simulink model "SIMULINK_U_a_C"  (R2023b)
settings: Solver=FixedStepAuto  StartTime=0.0  StopTime=sim_end_time  FixedStep=fixed_step_size  RelTol=1e-3
undefined symbols (not defined in the file): a, act_end, b, battery_threshold, bb, draw_gif, droneyeeUAV2_NUM, droneyeeUAV3_NUM, droneyeeUAV4_NUM, droneyeeUAV5_NUM, fixed_step_size, k, KD_x, KD_y, kd_z, KDD_x, KDD_y, KI_x, KI_y, ki_z, KII_x, KII_y, KP_x, KP_y, kp_z, KPP_x, KPP_y, lmt, omega, R, sim_end_time, uav10num, uav1num, uav2num, uav3num, uav4num, uav5num, uav6num, uav7num, uav8num, uav9num, UAV_NUM, Vel_Switch_1, Vel_Switch_10, Vel_Switch_11, Vel_Switch_12, Vel_Switch_13, Vel_Switch_14, Vel_Switch_15, Vel_Switch_16, Vel_Switch_17, Vel_Switch_18, Vel_Switch_19, Vel_Switch_2, Vel_Switch_20, Vel_Switch_3, Vel_Switch_4, Vel_Switch_5, Vel_Switch_6, Vel_Switch_7 ... (+11)
libraries: simulink x120, aerolibanimutils x1
(part 5 of 10)

== system SIMULINK_U_a_C/CMD_car1/CMD6 ==
  "clock " : Inport
  droneyeeUAV_states : Inport  Port=2
  droneyeeUAV_bat : Inport  Port=3
  Bus Selector : BusSelector  OutputSignals=x,y,z
  Constant : Constant  Value=sim_end_time
  Constant1 : Constant  Value=battery_threshold
  Constant2 : Constant  Value=z_d_for_land
  Constant3 : Constant  Value=0
  Constant4 : Constant  Value=UAV_NUM
  MATLAB Function1 : MATLAB Function  TreatAsAtomicUnit=on
  Manual Switch2 : ManualSwitch
  Sine Wave2 : Sin  Amplitude=0.3  Frequency=1.0
  Slider Gain3 : simulink/Math Operations/Slider Gain  gain=1  low=0  high=2
  Subsystem : Subsystem
  x_d : Outport  VectorParamsAs1DForOutWhenUnconnected=off
  y_d : Outport  Port=2  VectorParamsAs1DForOutWhenUnconnected=off
  z_d : Outport  Port=3  VectorParamsAs1DForOutWhenUnconnected=off
  yaw_d : Outport  Port=4  VectorParamsAs1DForOutWhenUnconnected=off
  wires:
  Manual Switch2/1 -> Slider Gain3/1
  Slider Gain3/1 -> yaw_d/1
  Sine Wave2/1 -> Manual Switch2/2
  Constant3/1 -> Manual Switch2/1
  MATLAB Function1/2(y_d_) -> y_d/1
  Constant2/1 -> MATLAB Function1/11(z_d_for_land)
  Subsystem/3(zd) -> MATLAB Function1/3(z_d)
  Constant1/1 -> MATLAB Function1/10(battery_threshold)
  MATLAB Function1/3(z_d_) -> z_d/1
  droneyeeUAV_states/1 -> Subsystem/2(uavstates), Bus Selector/1
  MATLAB Function1/1(x_d_) -> x_d/1
  Constant4/1 -> MATLAB Function1/12(UAV_NUM)
  Constant/1 -> MATLAB Function1/9(sim_time_end)
  Subsystem/1("xd ") -> MATLAB Function1/1(x_d)
  Subsystem/2(yd) -> MATLAB Function1/2(y_d)
  "clock "/1 -> Subsystem/1(clock), MATLAB Function1/4(timestamp)
  droneyeeUAV_bat/1 -> MATLAB Function1/8(battery_status)
  Bus Selector/1 -> MATLAB Function1/5(x)  "<x>"
  Bus Selector/2 -> MATLAB Function1/6(y)  "<y>"
  Bus Selector/3 -> MATLAB Function1/7(z)  "<z>"

== system SIMULINK_U_a_C/CMD_car1/CMD7 ==
  "clock " : Inport
  droneyeeUAV_states : Inport  Port=2
  droneyeeUAV_bat : Inport  Port=3
  Bus Selector : BusSelector  OutputSignals=x,y,z
  Constant : Constant  Value=sim_end_time
  Constant1 : Constant  Value=battery_threshold
  Constant2 : Constant  Value=z_d_for_land
  Constant3 : Constant  Value=0
  Constant4 : Constant  Value=UAV_NUM
  MATLAB Function1 : MATLAB Function  TreatAsAtomicUnit=on
  Manual Switch2 : ManualSwitch
  Sine Wave2 : Sin  Amplitude=0.3  Frequency=1.0
  Slider Gain3 : simulink/Math Operations/Slider Gain  gain=1  low=0  high=2
  Subsystem : Subsystem
  Terminator : Terminator
  x_d : Outport  VectorParamsAs1DForOutWhenUnconnected=off
  y_d : Outport  Port=2  VectorParamsAs1DForOutWhenUnconnected=off
  z_d : Outport  Port=3  VectorParamsAs1DForOutWhenUnconnected=off
  yaw_d : Outport  Port=4  VectorParamsAs1DForOutWhenUnconnected=off
  wires:
  Manual Switch2/1 -> Slider Gain3/1
  Slider Gain3/1 -> yaw_d/1
  Sine Wave2/1 -> Manual Switch2/2
  Constant3/1 -> Manual Switch2/1
  Bus Selector/1 -> MATLAB Function1/5(x)  "<x>"
  MATLAB Function1/2(y_d_) -> y_d/1
  Constant2/1 -> MATLAB Function1/11(z_d_for_land)
  Subsystem/3(zd) -> MATLAB Function1/3(z_d)
  Bus Selector/2 -> MATLAB Function1/6(y)  "<y>"
  Constant1/1 -> MATLAB Function1/10(battery_threshold)
  MATLAB Function1/3(z_d_) -> z_d/1
  MATLAB Function1/1(x_d_) -> x_d/1
  Constant4/1 -> MATLAB Function1/12(UAV_NUM)
  Bus Selector/3 -> MATLAB Function1/7(z)  "<z>"
  Constant/1 -> MATLAB Function1/9(sim_time_end)
  Subsystem/1("xd ") -> MATLAB Function1/1(x_d)
  Subsystem/2(yd) -> MATLAB Function1/2(y_d)
  "clock "/1 -> Subsystem/1(clock), MATLAB Function1/4(timestamp)
  droneyeeUAV_bat/1 -> MATLAB Function1/8(battery_status)
  droneyeeUAV_states/1 -> Subsystem/2(uavstates), Bus Selector/1

== system SIMULINK_U_a_C/CMD_car1/CMD8 ==
  "clock " : Inport
  droneyeeUAV_states : Inport  Port=2
  droneyeeUAV_bat : Inport  Port=3
  Bus Selector : BusSelector  OutputSignals=x,y,z
  Constant : Constant  Value=sim_end_time
  Constant1 : Constant  Value=battery_threshold
  Constant2 : Constant  Value=z_d_for_land
  Constant3 : Constant  Value=0
  Constant4 : Constant  Value=UAV_NUM
  MATLAB Function1 : MATLAB Function  TreatAsAtomicUnit=on
  Manual Switch2 : ManualSwitch
  Sine Wave2 : Sin  Amplitude=0.3  Frequency=1.0
  Slider Gain3 : simulink/Math Operations/Slider Gain  gain=1  low=0  high=2
  Subsystem : Subsystem
  x_d : Outport  VectorParamsAs1DForOutWhenUnconnected=off
  y_d : Outport  Port=2  VectorParamsAs1DForOutWhenUnconnected=off
  z_d : Outport  Port=3  VectorParamsAs1DForOutWhenUnconnected=off
  yaw_d : Outport  Port=4  VectorParamsAs1DForOutWhenUnconnected=off
  wires:
  Manual Switch2/1 -> Slider Gain3/1
  Slider Gain3/1 -> yaw_d/1
  Sine Wave2/1 -> Manual Switch2/2
  Constant3/1 -> Manual Switch2/1
  MATLAB Function1/2(y_d_) -> y_d/1
  Constant2/1 -> MATLAB Function1/11(z_d_for_land)
  Subsystem/3(zd) -> MATLAB Function1/3(z_d)
  Constant1/1 -> MATLAB Function1/10(battery_threshold)
  MATLAB Function1/3(z_d_) -> z_d/1
  droneyeeUAV_states/1 -> Subsystem/2(uavstates), Bus Selector/1
  MATLAB Function1/1(x_d_) -> x_d/1
  Constant4/1 -> MATLAB Function1/12(UAV_NUM)
  Constant/1 -> MATLAB Function1/9(sim_time_end)
  Subsystem/1("xd ") -> MATLAB Function1/1(x_d)
  Subsystem/2(yd) -> MATLAB Function1/2(y_d)
  "clock "/1 -> Subsystem/1(clock), MATLAB Function1/4(timestamp)
  droneyeeUAV_bat/1 -> MATLAB Function1/8(battery_status)
  Bus Selector/1 -> MATLAB Function1/5(x)  "<x>"
  Bus Selector/2 -> MATLAB Function1/6(y)  "<y>"
  Bus Selector/3 -> MATLAB Function1/7(z)  "<z>"

== system SIMULINK_U_a_C/CMD_car1/CMD9 ==
  "clock " : Inport
  droneyeeUAV_states : Inport  Port=2
  droneyeeUAV_bat : Inport  Port=3
  Bus Selector : BusSelector  OutputSignals=x,y,z
  Constant : Constant  Value=sim_end_time
  Constant1 : Constant  Value=battery_threshold
  Constant2 : Constant  Value=z_d_for_land
  Constant3 : Constant  Value=0
  Constant4 : Constant  Value=UAV_NUM
  MATLAB Function1 : MATLAB Function  TreatAsAtomicUnit=on
  Manual Switch2 : ManualSwitch
  Sine Wave2 : Sin  Amplitude=0.3  Frequency=1.0
  Slider Gain3 : simulink/Math Operations/Slider Gain  gain=1  low=0  high=2
  Subsystem : Subsystem
  Terminator : Terminator
  x_d : Outport  VectorParamsAs1DForOutWhenUnconnected=off
  y_d : Outport  Port=2  VectorParamsAs1DForOutWhenUnconnected=off
  z_d : Outport  Port=3  VectorParamsAs1DForOutWhenUnconnected=off
  yaw_d : Outport  Port=4  VectorParamsAs1DForOutWhenUnconnected=off
  wires:
  Manual Switch2/1 -> Slider Gain3/1
  Slider Gain3/1 -> yaw_d/1
  Sine Wave2/1 -> Manual Switch2/2
  Constant3/1 -> Manual Switch2/1
  Bus Selector/1 -> MATLAB Function1/5(x)  "<x>"
  MATLAB Function1/2(y_d_) -> y_d/1
  Constant2/1 -> MATLAB Function1/11(z_d_for_land)
  Subsystem/3(zd) -> MATLAB Function1/3(z_d)
  Bus Selector/2 -> MATLAB Function1/6(y)  "<y>"
  Constant1/1 -> MATLAB Function1/10(battery_threshold)
  MATLAB Function1/3(z_d_) -> z_d/1
  MATLAB Function1/1(x_d_) -> x_d/1
  Constant4/1 -> MATLAB Function1/12(UAV_NUM)
  Bus Selector/3 -> MATLAB Function1/7(z)  "<z>"
  Constant/1 -> MATLAB Function1/9(sim_time_end)
  Subsystem/1("xd ") -> MATLAB Function1/1(x_d)
  Subsystem/2(yd) -> MATLAB Function1/2(y_d)
  "clock "/1 -> Subsystem/1(clock), MATLAB Function1/4(timestamp)
  droneyeeUAV_bat/1 -> MATLAB Function1/8(battery_status)
  droneyeeUAV_states/1 -> Subsystem/2(uavstates), Bus Selector/1

== system SIMULINK_U_a_C/control system_UAV/Baseline Controller1 ==
  X_e : Inport
  Y_e : Inport  Port=2
  " Z_e " : Inport  Port=3
  Yaw_e : Inport  Port=4
  " V_x" : Inport  Port=5
  V_y : Inport  Port=6
  "V_z " : Inport  Port=7
  x_d : Inport  Port=8
  y_d : Inport  Port=9
  Z_d : Inport  Port=10
  Yaw_d : Inport  Port=11
  Constant : Constant  Commented=on  Value=omega*R*2
  Demux : Demux  Outputs=2
  Heading controller : Subsystem
  "Height controller " : Subsystem
  MATLAB Function : MATLAB Function  Commented=on  TreatAsAtomicUnit=on
  Position controller : Subsystem
  Saturation1 : Saturate  UpperLimit=lmt  LowerLimit=-lmt
  Saturation2 : Saturate  UpperLimit=lmt  LowerLimit=-lmt
  ux : Outport  VectorParamsAs1DForOutWhenUnconnected=off
  uy : Outport  Port=2  VectorParamsAs1DForOutWhenUnconnected=off
  Z_velocity_d. [-1,1] : Outport  Port=3  VectorParamsAs1DForOutWhenUnconnected=off
  yaw_rate_d [-1,1] : Outport  Port=4  VectorParamsAs1DForOutWhenUnconnected=off
  wires:
  " Z_e "/1 -> "Height controller "/2(Z_e (m))
  X_e/1 -> Position controller/1(X_e (m))
  Y_e/1 -> Position controller/2(Y_e (m))
  Yaw_d/1 -> Heading controller/2(yaw_d. (rad))
  Demux/1 -> ux/1
  Demux/2 -> uy/1
  Constant/1 -> MATLAB Function/2(a)
  Z_d/1 -> "Height controller "/1(Z_d. (m))
  x_d/1 -> Position controller/3(X_d (m))
  y_d/1 -> Position controller/4(Y_d (m))
  Yaw_e/1 -> Heading controller/1(yaw_e (rad))  "yaw"
  "V_z "/1 -> "Height controller "/3(V_z)
  Heading controller/1(yaw_rate_d. (rad/s)) -> yaw_rate_d [-1,1]/1
  "Height controller "/1(Z_velocity_d (m/s)) -> Saturation2/1
  Saturation1/1 -> Demux/1
  Position controller/1(uxy) -> Saturation1/1
  Saturation2/1 -> Z_velocity_d. [-1,1]/1

== system SIMULINK_U_a_C/control system_UAV/Baseline Controller10 ==
  X_e : Inport
  Y_e : Inport  Port=2
  " Z_e " : Inport  Port=3
  Yaw_e : Inport  Port=4
  " V_x" : Inport  Port=5
  V_y : Inport  Port=6
  "V_z " : Inport  Port=7
  x_d : Inport  Port=8
  y_d : Inport  Port=9
  Z_d : Inport  Port=10
  Yaw_d : Inport  Port=11
  Demux : Demux  Outputs=2
  Heading controller : Subsystem
  "Height controller " : Subsystem
  Position controller : Subsystem
  Saturation : Saturate  UpperLimit=lmt  LowerLimit=-lmt
  Saturation1 : Saturate  UpperLimit=lmt  LowerLimit=-lmt
  Saturation2 : Saturate  UpperLimit=lmt  LowerLimit=-lmt
  Scope : Scope
  ux : Outport  VectorParamsAs1DForOutWhenUnconnected=off
  uy : Outport  Port=2  VectorParamsAs1DForOutWhenUnconnected=off
  Z_velocity_d. [-1,1] : Outport  Port=3  VectorParamsAs1DForOutWhenUnconnected=off
  yaw_rate_d [-1,1] : Outport  Port=4  VectorParamsAs1DForOutWhenUnconnected=off
  wires:
  X_e/1 -> Position controller/1(X_e (m))
  Y_e/1 -> Position controller/2(Y_e (m))
  Yaw_d/1 -> Heading controller/2(yaw_d. (rad))
  Saturation/1 -> Demux/1
  Demux/1 -> Scope/1, ux/1
  Demux/2 -> uy/1
  x_d/1 -> Position controller/3(X_d (m))
  y_d/1 -> Position controller/4(Y_d (m))
  Yaw_e/1 -> Heading controller/1(yaw_e (rad))  "yaw"
  Position controller/1(uxy) -> Saturation/1
  Z_d/1 -> "Height controller "/1(Z_d. (m))
  " Z_e "/1 -> "Height controller "/2(Z_e (m))
  "Height controller "/1(Z_velocity_d (m/s)) -> Saturation2/1
  "V_z "/1 -> "Height controller "/3(V_z)
  Saturation2/1 -> Z_velocity_d. [-1,1]/1

== system SIMULINK_U_a_C/control system_UAV/Baseline Controller2 ==
  X_e : Inport
  Y_e : Inport  Port=2
  " Z_e " : Inport  Port=3
  Yaw_e : Inport  Port=4
  " V_x" : Inport  Port=5
  V_y : Inport  Port=6
  "V_z " : Inport  Port=7
  x_d : Inport  Port=8
  y_d : Inport  Port=9
  Z_d : Inport  Port=10
  Yaw_d : Inport  Port=11
  Constant : Constant  Commented=on  Value=omega*R*2
  Demux : Demux  Outputs=2
  Heading controller : Subsystem
  "Height controller " : Subsystem
  MATLAB Function : MATLAB Function  Commented=on  TreatAsAtomicUnit=on
  Position controller : Subsystem
  Saturation : Saturate  UpperLimit=lmt  LowerLimit=-lmt
  Saturation1 : Saturate  UpperLimit=lmt  LowerLimit=-lmt
  ux : Outport  VectorParamsAs1DForOutWhenUnconnected=off
  uy : Outport  Port=2  VectorParamsAs1DForOutWhenUnconnected=off
  Z_velocity_d. [-1,1] : Outport  Port=3  VectorParamsAs1DForOutWhenUnconnected=off
  yaw_rate_d [-1,1] : Outport  Port=4  VectorParamsAs1DForOutWhenUnconnected=off
  wires:
  Position controller/1(uxy) -> Saturation/1
  Yaw_e/1 -> Heading controller/1(yaw_e (rad))  "yaw"
  y_d/1 -> Position controller/4(Y_d (m))
  x_d/1 -> Position controller/3(X_d (m))
  Constant/1 -> MATLAB Function/2(a)
  Demux/2 -> uy/1
  Demux/1 -> ux/1
  Saturation/1 -> Demux/1
  Yaw_d/1 -> Heading controller/2(yaw_d. (rad))
  Y_e/1 -> Position controller/2(Y_e (m))
  X_e/1 -> Position controller/1(X_e (m))
  Z_d/1 -> "Height controller "/1(Z_d. (m))
  " Z_e "/1 -> "Height controller "/2(Z_e (m))
  "V_z "/1 -> "Height controller "/3(V_z)
  Saturation1/1 -> Z_velocity_d. [-1,1]/1
  "Height controller "/1(Z_velocity_d (m/s)) -> Saturation1/1

== system SIMULINK_U_a_C/control system_UAV/Baseline Controller3 ==
  X_e : Inport
  Y_e : Inport  Port=2
  " Z_e " : Inport  Port=3
  Yaw_e : Inport  Port=4
  " V_x" : Inport  Port=5
  V_y : Inport  Port=6
  "V_z " : Inport  Port=7
  x_d : Inport  Port=8
  y_d : Inport  Port=9
  Z_d : Inport  Port=10
  Yaw_d : Inport  Port=11
  Constant : Constant  Commented=on  Value=omega*R*2
  Demux : Demux  Outputs=2
  Heading controller : Subsystem
  "Height controller " : Subsystem
  MATLAB Function : MATLAB Function  Commented=on  TreatAsAtomicUnit=on
  Position controller : Subsystem
  Saturation : Saturate  UpperLimit=lmt  LowerLimit=-lmt
  Saturation1 : Saturate  UpperLimit=lmt  LowerLimit=-lmt
  ux : Outport  VectorParamsAs1DForOutWhenUnconnected=off
  uy : Outport  Port=2  VectorParamsAs1DForOutWhenUnconnected=off
  Z_velocity_d. [-1,1] : Outport  Port=3  VectorParamsAs1DForOutWhenUnconnected=off
  yaw_rate_d [-1,1] : Outport  Port=4  VectorParamsAs1DForOutWhenUnconnected=off
  wires:
  X_e/1 -> Position controller/1(X_e (m))
  Y_e/1 -> Position controller/2(Y_e (m))
  Yaw_d/1 -> Heading controller/2(yaw_d. (rad))
  Saturation/1 -> Demux/1
  Demux/1 -> ux/1
  Demux/2 -> uy/1
  Constant/1 -> MATLAB Function/2(a)
  x_d/1 -> Position controller/3(X_d (m))
  y_d/1 -> Position controller/4(Y_d (m))
  Yaw_e/1 -> Heading controller/1(yaw_e (rad))  "yaw"
  Position controller/1(uxy) -> Saturation/1
  "Height controller "/1(Z_velocity_d (m/s)) -> Saturation1/1
  " Z_e "/1 -> "Height controller "/2(Z_e (m))
  "V_z "/1 -> "Height controller "/3(V_z)
  Z_d/1 -> "Height controller "/1(Z_d. (m))
  Saturation1/1 -> Z_velocity_d. [-1,1]/1

== system SIMULINK_U_a_C/control system_UAV/Baseline Controller4 ==
  X_e : Inport
  Y_e : Inport  Port=2
  " Z_e " : Inport  Port=3
  Yaw_e : Inport  Port=4
  " V_x" : Inport  Port=5
  V_y : Inport  Port=6
  "V_z " : Inport  Port=7
  x_d : Inport  Port=8
  y_d : Inport  Port=9
  Z_d : Inport  Port=10
  Yaw_d : Inport  Port=11
  Constant : Constant  Commented=on  Value=omega*R*2
  Demux : Demux  Outputs=2
  Heading controller : Subsystem
  "Height controller " : Subsystem
  MATLAB Function : MATLAB Function  Commented=on  TreatAsAtomicUnit=on
  Position controller : Subsystem
  Saturation : Saturate  UpperLimit=lmt  LowerLimit=-lmt
  Saturation1 : Saturate  UpperLimit=lmt  LowerLimit=-lmt
  ux : Outport  VectorParamsAs1DForOutWhenUnconnected=off
  uy : Outport  Port=2  VectorParamsAs1DForOutWhenUnconnected=off
  Z_velocity_d. [-1,1] : Outport  Port=3  VectorParamsAs1DForOutWhenUnconnected=off
  yaw_rate_d [-1,1] : Outport  Port=4  VectorParamsAs1DForOutWhenUnconnected=off
  wires:
  Position controller/1(uxy) -> Saturation/1
  Yaw_e/1 -> Heading controller/1(yaw_e (rad))  "yaw"
  y_d/1 -> Position controller/4(Y_d (m))
  x_d/1 -> Position controller/3(X_d (m))
  Constant/1 -> MATLAB Function/2(a)
  Demux/2 -> uy/1
  Demux/1 -> ux/1
  Saturation/1 -> Demux/1
  Yaw_d/1 -> Heading controller/2(yaw_d. (rad))
  Y_e/1 -> Position controller/2(Y_e (m))
  X_e/1 -> Position controller/1(X_e (m))
  Z_d/1 -> "Height controller "/1(Z_d. (m))
  " Z_e "/1 -> "Height controller "/2(Z_e (m))
  Saturation1/1 -> Z_velocity_d. [-1,1]/1
  "Height controller "/1(Z_velocity_d (m/s)) -> Saturation1/1
  "V_z "/1 -> "Height controller "/3(V_z)

== system SIMULINK_U_a_C/control system_UAV/Baseline Controller5 ==
  X_e : Inport
  Y_e : Inport  Port=2
  " Z_e " : Inport  Port=3
  Yaw_e : Inport  Port=4
  " V_x" : Inport  Port=5
  V_y : Inport  Port=6
  "V_z " : Inport  Port=7
  x_d : Inport  Port=8
  y_d : Inport  Port=9
  Z_d : Inport  Port=10
  Yaw_d : Inport  Port=11
  Demux : Demux  Outputs=2
  Heading controller : Subsystem
  "Height controller " : Subsystem
  Position controller : Subsystem
  Saturation : Saturate  UpperLimit=lmt  LowerLimit=-lmt
  Saturation1 : Saturate  UpperLimit=lmt  LowerLimit=-lmt
  Saturation2 : Saturate  UpperLimit=lmt  LowerLimit=-lmt
  Scope : Scope
  ux : Outport  VectorParamsAs1DForOutWhenUnconnected=off
  uy : Outport  Port=2  VectorParamsAs1DForOutWhenUnconnected=off
  Z_velocity_d. [-1,1] : Outport  Port=3  VectorParamsAs1DForOutWhenUnconnected=off
  yaw_rate_d [-1,1] : Outport  Port=4  VectorParamsAs1DForOutWhenUnconnected=off
  wires:
  X_e/1 -> Position controller/1(X_e (m))
  Y_e/1 -> Position controller/2(Y_e (m))
  Yaw_d/1 -> Heading controller/2(yaw_d. (rad))
  Saturation/1 -> Demux/1
  Demux/1 -> Scope/1, ux/1
  Demux/2 -> uy/1
  x_d/1 -> Position controller/3(X_d (m))
  y_d/1 -> Position controller/4(Y_d (m))
  Yaw_e/1 -> Heading controller/1(yaw_e (rad))  "yaw"
  Position controller/1(uxy) -> Saturation/1
  Z_d/1 -> "Height controller "/1(Z_d. (m))
  " Z_e "/1 -> "Height controller "/2(Z_e (m))
  "Height controller "/1(Z_velocity_d (m/s)) -> Saturation2/1
  "V_z "/1 -> "Height controller "/3(V_z)
  Saturation2/1 -> Z_velocity_d. [-1,1]/1

== system SIMULINK_U_a_C/control system_UAV/Baseline Controller6 ==
  X_e : Inport
  Y_e : Inport  Port=2
  " Z_e " : Inport  Port=3
  Yaw_e : Inport  Port=4
  " V_x" : Inport  Port=5
  V_y : Inport  Port=6
  "V_z " : Inport  Port=7
  x_d : Inport  Port=8
  y_d : Inport  Port=9
  Z_d : Inport  Port=10
  Yaw_d : Inport  Port=11
  Demux : Demux  Outputs=2
  Heading controller : Subsystem
  "Height controller " : Subsystem
  Position controller : Subsystem
  Saturation : Saturate  UpperLimit=lmt  LowerLimit=-lmt
  Saturation1 : Saturate  UpperLimit=lmt  LowerLimit=-lmt
  Saturation2 : Saturate  UpperLimit=lmt  LowerLimit=-lmt
  Scope : Scope
  ux : Outport  VectorParamsAs1DForOutWhenUnconnected=off
  uy : Outport  Port=2  VectorParamsAs1DForOutWhenUnconnected=off
  Z_velocity_d. [-1,1] : Outport  Port=3  VectorParamsAs1DForOutWhenUnconnected=off
  yaw_rate_d [-1,1] : Outport  Port=4  VectorParamsAs1DForOutWhenUnconnected=off
  wires:
  X_e/1 -> Position controller/1(X_e (m))
  Y_e/1 -> Position controller/2(Y_e (m))
  Yaw_d/1 -> Heading controller/2(yaw_d. (rad))
  Saturation/1 -> Demux/1
  Demux/1 -> Scope/1, ux/1
  Demux/2 -> uy/1
  x_d/1 -> Position controller/3(X_d (m))
  y_d/1 -> Position controller/4(Y_d (m))
  Yaw_e/1 -> Heading controller/1(yaw_e (rad))  "yaw"
  Position controller/1(uxy) -> Saturation/1
  Z_d/1 -> "Height controller "/1(Z_d. (m))
  " Z_e "/1 -> "Height controller "/2(Z_e (m))
  "Height controller "/1(Z_velocity_d (m/s)) -> Saturation2/1
  "V_z "/1 -> "Height controller "/3(V_z)
  Saturation2/1 -> Z_velocity_d. [-1,1]/1

== system SIMULINK_U_a_C/control system_UAV/Baseline Controller7 ==
  X_e : Inport
  Y_e : Inport  Port=2
  " Z_e " : Inport  Port=3
  Yaw_e : Inport  Port=4
  " V_x" : Inport  Port=5
  V_y : Inport  Port=6
  "V_z " : Inport  Port=7
  x_d : Inport  Port=8
  y_d : Inport  Port=9
  Z_d : Inport  Port=10
  Yaw_d : Inport  Port=11
  Demux : Demux  Outputs=2
  Heading controller : Subsystem
  "Height controller " : Subsystem
  Position controller : Subsystem
  Saturation : Saturate  UpperLimit=lmt  LowerLimit=-lmt
  Saturation1 : Saturate  UpperLimit=lmt  LowerLimit=-lmt
  Saturation2 : Saturate  UpperLimit=lmt  LowerLimit=-lmt
  Scope : Scope
  ux : Outport  VectorParamsAs1DForOutWhenUnconnected=off
  uy : Outport  Port=2  VectorParamsAs1DForOutWhenUnconnected=off
  Z_velocity_d. [-1,1] : Outport  Port=3  VectorParamsAs1DForOutWhenUnconnected=off
  yaw_rate_d [-1,1] : Outport  Port=4  VectorParamsAs1DForOutWhenUnconnected=off
  wires:
  X_e/1 -> Position controller/1(X_e (m))
  Y_e/1 -> Position controller/2(Y_e (m))
  Yaw_d/1 -> Heading controller/2(yaw_d. (rad))
  Saturation/1 -> Demux/1
  Demux/1 -> Scope/1, ux/1
  Demux/2 -> uy/1
  x_d/1 -> Position controller/3(X_d (m))
  y_d/1 -> Position controller/4(Y_d (m))
  Yaw_e/1 -> Heading controller/1(yaw_e (rad))  "yaw"
  Position controller/1(uxy) -> Saturation/1
  Z_d/1 -> "Height controller "/1(Z_d. (m))
  " Z_e "/1 -> "Height controller "/2(Z_e (m))
  "Height controller "/1(Z_velocity_d (m/s)) -> Saturation2/1
  "V_z "/1 -> "Height controller "/3(V_z)
  Saturation2/1 -> Z_velocity_d. [-1,1]/1

== system SIMULINK_U_a_C/control system_UAV/Baseline Controller8 ==
  X_e : Inport
  Y_e : Inport  Port=2
  " Z_e " : Inport  Port=3
  Yaw_e : Inport  Port=4
  " V_x" : Inport  Port=5
  V_y : Inport  Port=6
  "V_z " : Inport  Port=7
  x_d : Inport  Port=8
  y_d : Inport  Port=9
  Z_d : Inport  Port=10
  Yaw_d : Inport  Port=11
  Demux : Demux  Outputs=2
  Heading controller : Subsystem
  "Height controller " : Subsystem
  Position controller : Subsystem
  Saturation : Saturate  UpperLimit=lmt  LowerLimit=-lmt
  Saturation1 : Saturate  UpperLimit=lmt  LowerLimit=-lmt
  Saturation2 : Saturate  UpperLimit=lmt  LowerLimit=-lmt
  Scope : Scope
  ux : Outport  VectorParamsAs1DForOutWhenUnconnected=off
  uy : Outport  Port=2  VectorParamsAs1DForOutWhenUnconnected=off
  Z_velocity_d. [-1,1] : Outport  Port=3  VectorParamsAs1DForOutWhenUnconnected=off
  yaw_rate_d [-1,1] : Outport  Port=4  VectorParamsAs1DForOutWhenUnconnected=off
  wires:
  X_e/1 -> Position controller/1(X_e (m))
  Y_e/1 -> Position controller/2(Y_e (m))
  Yaw_d/1 -> Heading controller/2(yaw_d. (rad))
  Saturation/1 -> Demux/1
  Demux/1 -> Scope/1, ux/1
  Demux/2 -> uy/1
  x_d/1 -> Position controller/3(X_d (m))
  y_d/1 -> Position controller/4(Y_d (m))
  Yaw_e/1 -> Heading controller/1(yaw_e (rad))  "yaw"
  Position controller/1(uxy) -> Saturation/1
  Z_d/1 -> "Height controller "/1(Z_d. (m))
  " Z_e "/1 -> "Height controller "/2(Z_e (m))
  "Height controller "/1(Z_velocity_d (m/s)) -> Saturation2/1
  "V_z "/1 -> "Height controller "/3(V_z)
  Saturation2/1 -> Z_velocity_d. [-1,1]/1

== system SIMULINK_U_a_C/control system_UAV/Baseline Controller9 ==
  X_e : Inport
  Y_e : Inport  Port=2
  " Z_e " : Inport  Port=3
  Yaw_e : Inport  Port=4
  " V_x" : Inport  Port=5
  V_y : Inport  Port=6
  "V_z " : Inport  Port=7
  x_d : Inport  Port=8
  y_d : Inport  Port=9
  Z_d : Inport  Port=10
  Yaw_d : Inport  Port=11
  Demux : Demux  Outputs=2
  Heading controller : Subsystem
  "Height controller " : Subsystem
  Position controller : Subsystem
  Saturation : Saturate  UpperLimit=lmt  LowerLimit=-lmt
  Saturation1 : Saturate  UpperLimit=lmt  LowerLimit=-lmt
  Saturation2 : Saturate  UpperLimit=lmt  LowerLimit=-lmt
  Scope : Scope
  ux : Outport  VectorParamsAs1DForOutWhenUnconnected=off
  uy : Outport  Port=2  VectorParamsAs1DForOutWhenUnconnected=off
  Z_velocity_d. [-1,1] : Outport  Port=3  VectorParamsAs1DForOutWhenUnconnected=off
  yaw_rate_d [-1,1] : Outport  Port=4  VectorParamsAs1DForOutWhenUnconnected=off
  wires:
  X_e/1 -> Position controller/1(X_e (m))
  Y_e/1 -> Position controller/2(Y_e (m))
  Yaw_d/1 -> Heading controller/2(yaw_d. (rad))
  Saturation/1 -> Demux/1
  Demux/1 -> Scope/1, ux/1
  Demux/2 -> uy/1
  x_d/1 -> Position controller/3(X_d (m))
  y_d/1 -> Position controller/4(Y_d (m))
  Yaw_e/1 -> Heading controller/1(yaw_e (rad))  "yaw"
  Position controller/1(uxy) -> Saturation/1
  Z_d/1 -> "Height controller "/1(Z_d. (m))
  " Z_e "/1 -> "Height controller "/2(Z_e (m))
  "Height controller "/1(Z_velocity_d (m/s)) -> Saturation2/1
  "V_z "/1 -> "Height controller "/3(V_z)
  Saturation2/1 -> Z_velocity_d. [-1,1]/1

== system SIMULINK_U_a_C/control system_car1/Baseline Controller1 ==
  X_e : Inport
  Y_e : Inport  Port=2
  " Z_e " : Inport  Port=3
  Yaw_e : Inport  Port=4
  " V_x" : Inport  Port=5
  V_y : Inport  Port=6
  "V_z " : Inport  Port=7
  x_d : Inport  Port=8
  y_d : Inport  Port=9
  Z_d : Inport  Port=10
  Yaw_d : Inport  Port=11
  Constant : Constant  Commented=on  Value=omega*R*2
  Constant1 : Constant  Value=0
  Demux : Demux  Outputs=2
  Heading controller : Subsystem
  "Height controller " : Subsystem
  MATLAB Function : MATLAB Function  Commented=on  TreatAsAtomicUnit=on
  Position controller : Subsystem
  Saturation1 : Saturate  UpperLimit=lmt  LowerLimit=-lmt
  Saturation2 : Saturate  UpperLimit=lmt  LowerLimit=-lmt
  Terminator : Terminator
  ux : Outport  VectorParamsAs1DForOutWhenUnconnected=off
  uy : Outport  Port=2  VectorParamsAs1DForOutWhenUnconnected=off
  Z_velocity_d. [-1,1] : Outport  Port=3  VectorParamsAs1DForOutWhenUnconnected=off
  yaw_rate_d [-1,1] : Outport  Port=4  VectorParamsAs1DForOutWhenUnconnected=off
  wires:
  " Z_e "/1 -> "Height controller "/2(Z_e (m))
  X_e/1 -> Position controller/1(X_e (m))
  Y_e/1 -> Position controller/2(Y_e (m))
  Yaw_d/1 -> Heading controller/2(yaw_d. (rad))
  Demux/1 -> ux/1
  Demux/2 -> uy/1
  Constant/1 -> MATLAB Function/2(a)
  Z_d/1 -> "Height controller "/1(Z_d. (m))
  x_d/1 -> Position controller/3(X_d (m))
  y_d/1 -> Position controller/4(Y_d (m))
  Yaw_e/1 -> Heading controller/1(yaw_e (rad))  "yaw"
  "V_z "/1 -> "Height controller "/3(V_z)
  Heading controller/1(yaw_rate_d. (rad/s)) -> yaw_rate_d [-1,1]/1
  "Height controller "/1(Z_velocity_d (m/s)) -> Saturation2/1
  Saturation1/1 -> Demux/1
  Position controller/1(uxy) -> Saturation1/1
  Constant1/1 -> Z_velocity_d. [-1,1]/1
  Saturation2/1 -> Terminator/1

== system SIMULINK_U_a_C/control system_car1/Baseline Controller10 ==
  X_e : Inport
  Y_e : Inport  Port=2
  " Z_e " : Inport  Port=3
  Yaw_e : Inport  Port=4
  " V_x" : Inport  Port=5
  V_y : Inport  Port=6
  "V_z " : Inport  Port=7
  x_d : Inport  Port=8
  y_d : Inport  Port=9
  Z_d : Inport  Port=10
  Yaw_d : Inport  Port=11
  Constant : Constant  Commented=on  Value=omega*R*2
  Constant1 : Constant  Value=0
  Demux : Demux  Outputs=2
  Heading controller : Subsystem
  "Height controller " : Subsystem
  MATLAB Function : MATLAB Function  Commented=on  TreatAsAtomicUnit=on
  Position controller : Subsystem
  Saturation1 : Saturate  UpperLimit=lmt  LowerLimit=-lmt
  Saturation2 : Saturate  UpperLimit=lmt  LowerLimit=-lmt
  Terminator : Terminator
  ux : Outport  VectorParamsAs1DForOutWhenUnconnected=off
  uy : Outport  Port=2  VectorParamsAs1DForOutWhenUnconnected=off
  Z_velocity_d. [-1,1] : Outport  Port=3  VectorParamsAs1DForOutWhenUnconnected=off
  yaw_rate_d [-1,1] : Outport  Port=4  VectorParamsAs1DForOutWhenUnconnected=off
  wires:
  " Z_e "/1 -> "Height controller "/2(Z_e (m))
  X_e/1 -> Position controller/1(X_e (m))
  Y_e/1 -> Position controller/2(Y_e (m))
  Yaw_d/1 -> Heading controller/2(yaw_d. (rad))
  Demux/1 -> ux/1
  Demux/2 -> uy/1
  Constant/1 -> MATLAB Function/2(a)
  Z_d/1 -> "Height controller "/1(Z_d. (m))
  x_d/1 -> Position controller/3(X_d (m))
  y_d/1 -> Position controller/4(Y_d (m))
  Yaw_e/1 -> Heading controller/1(yaw_e (rad))  "yaw"
  "V_z "/1 -> "Height controller "/3(V_z)
  Heading controller/1(yaw_rate_d. (rad/s)) -> yaw_rate_d [-1,1]/1
  "Height controller "/1(Z_velocity_d (m/s)) -> Saturation2/1
  Saturation1/1 -> Demux/1
  Position controller/1(uxy) -> Saturation1/1
  Constant1/1 -> Z_velocity_d. [-1,1]/1
  Saturation2/1 -> Terminator/1

== system SIMULINK_U_a_C/control system_car1/Baseline Controller2 ==
  X_e : Inport
  Y_e : Inport  Port=2
  " Z_e " : Inport  Port=3
  Yaw_e : Inport  Port=4
  " V_x" : Inport  Port=5
  V_y : Inport  Port=6
  "V_z " : Inport  Port=7
  x_d : Inport  Port=8
  y_d : Inport  Port=9
  Z_d : Inport  Port=10
  Yaw_d : Inport  Port=11
  Constant : Constant  Commented=on  Value=omega*R*2
  Constant1 : Constant  Value=0
  Demux : Demux  Outputs=2
  Heading controller : Subsystem
  "Height controller " : Subsystem
  MATLAB Function : MATLAB Function  Commented=on  TreatAsAtomicUnit=on
  Position controller : Subsystem
  Saturation1 : Saturate  UpperLimit=lmt  LowerLimit=-lmt
  Saturation2 : Saturate  UpperLimit=lmt  LowerLimit=-lmt
  Terminator : Terminator
  ux : Outport  VectorParamsAs1DForOutWhenUnconnected=off
  uy : Outport  Port=2  VectorParamsAs1DForOutWhenUnconnected=off
  Z_velocity_d. [-1,1] : Outport  Port=3  VectorParamsAs1DForOutWhenUnconnected=off
  yaw_rate_d [-1,1] : Outport  Port=4  VectorParamsAs1DForOutWhenUnconnected=off
  wires:
  " Z_e "/1 -> "Height controller "/2(Z_e (m))
  X_e/1 -> Position controller/1(X_e (m))
  Y_e/1 -> Position controller/2(Y_e (m))
  Yaw_d/1 -> Heading controller/2(yaw_d. (rad))
  Demux/1 -> ux/1
  Demux/2 -> uy/1
  Constant/1 -> MATLAB Function/2(a)
  Z_d/1 -> "Height controller "/1(Z_d. (m))
  x_d/1 -> Position controller/3(X_d (m))
  y_d/1 -> Position controller/4(Y_d (m))
  Yaw_e/1 -> Heading controller/1(yaw_e (rad))  "yaw"
  "V_z "/1 -> "Height controller "/3(V_z)
  Heading controller/1(yaw_rate_d. (rad/s)) -> yaw_rate_d [-1,1]/1
  "Height controller "/1(Z_velocity_d (m/s)) -> Saturation2/1
  Saturation1/1 -> Demux/1
  Position controller/1(uxy) -> Saturation1/1
  Constant1/1 -> Z_velocity_d. [-1,1]/1
  Saturation2/1 -> Terminator/1

== system SIMULINK_U_a_C/control system_car1/Baseline Controller3 ==
  X_e : Inport
  Y_e : Inport  Port=2
  " Z_e " : Inport  Port=3
  Yaw_e : Inport  Port=4
  " V_x" : Inport  Port=5
  V_y : Inport  Port=6
  "V_z " : Inport  Port=7
  x_d : Inport  Port=8
  y_d : Inport  Port=9
  Z_d : Inport  Port=10
  Yaw_d : Inport  Port=11
  Constant : Constant  Commented=on  Value=omega*R*2
  Constant1 : Constant  Value=0
  Demux : Demux  Outputs=2
  Heading controller : Subsystem
  "Height controller " : Subsystem
  MATLAB Function : MATLAB Function  Commented=on  TreatAsAtomicUnit=on
  Position controller : Subsystem
  Saturation1 : Saturate  UpperLimit=lmt  LowerLimit=-lmt
  Saturation2 : Saturate  UpperLimit=lmt  LowerLimit=-lmt
  Terminator : Terminator
  ux : Outport  VectorParamsAs1DForOutWhenUnconnected=off
  uy : Outport  Port=2  VectorParamsAs1DForOutWhenUnconnected=off
  Z_velocity_d. [-1,1] : Outport  Port=3  VectorParamsAs1DForOutWhenUnconnected=off
  yaw_rate_d [-1,1] : Outport  Port=4  VectorParamsAs1DForOutWhenUnconnected=off
  wires:
  " Z_e "/1 -> "Height controller "/2(Z_e (m))
  X_e/1 -> Position controller/1(X_e (m))
  Y_e/1 -> Position controller/2(Y_e (m))
  Yaw_d/1 -> Heading controller/2(yaw_d. (rad))
  Demux/1 -> ux/1
  Demux/2 -> uy/1
  Constant/1 -> MATLAB Function/2(a)
  Z_d/1 -> "Height controller "/1(Z_d. (m))
  x_d/1 -> Position controller/3(X_d (m))
  y_d/1 -> Position controller/4(Y_d (m))
  Yaw_e/1 -> Heading controller/1(yaw_e (rad))  "yaw"
  "V_z "/1 -> "Height controller "/3(V_z)
  Heading controller/1(yaw_rate_d. (rad/s)) -> yaw_rate_d [-1,1]/1
  "Height controller "/1(Z_velocity_d (m/s)) -> Saturation2/1
  Saturation1/1 -> Demux/1
  Position controller/1(uxy) -> Saturation1/1
  Constant1/1 -> Z_velocity_d. [-1,1]/1
  Saturation2/1 -> Terminator/1

== system SIMULINK_U_a_C/control system_car1/Baseline Controller4 ==
  X_e : Inport
  Y_e : Inport  Port=2
  " Z_e " : Inport  Port=3
  Yaw_e : Inport  Port=4
  " V_x" : Inport  Port=5
  V_y : Inport  Port=6
  "V_z " : Inport  Port=7
  x_d : Inport  Port=8
  y_d : Inport  Port=9
  Z_d : Inport  Port=10
  Yaw_d : Inport  Port=11
  Constant : Constant  Commented=on  Value=omega*R*2
  Constant1 : Constant  Value=0
  Demux : Demux  Outputs=2
  Heading controller : Subsystem
  "Height controller " : Subsystem
  MATLAB Function : MATLAB Function  Commented=on  TreatAsAtomicUnit=on
  Position controller : Subsystem
  Saturation1 : Saturate  UpperLimit=lmt  LowerLimit=-lmt
  Saturation2 : Saturate  UpperLimit=lmt  LowerLimit=-lmt
  Terminator : Terminator
  ux : Outport  VectorParamsAs1DForOutWhenUnconnected=off
  uy : Outport  Port=2  VectorParamsAs1DForOutWhenUnconnected=off
  Z_velocity_d. [-1,1] : Outport  Port=3  VectorParamsAs1DForOutWhenUnconnected=off
  yaw_rate_d [-1,1] : Outport  Port=4  VectorParamsAs1DForOutWhenUnconnected=off
  wires:
  " Z_e "/1 -> "Height controller "/2(Z_e (m))
  X_e/1 -> Position controller/1(X_e (m))
  Y_e/1 -> Position controller/2(Y_e (m))
  Yaw_d/1 -> Heading controller/2(yaw_d. (rad))
  Demux/1 -> ux/1
  Demux/2 -> uy/1
  Constant/1 -> MATLAB Function/2(a)
  Z_d/1 -> "Height controller "/1(Z_d. (m))
  x_d/1 -> Position controller/3(X_d (m))
  y_d/1 -> Position controller/4(Y_d (m))
  Yaw_e/1 -> Heading controller/1(yaw_e (rad))  "yaw"
  "V_z "/1 -> "Height controller "/3(V_z)
  Heading controller/1(yaw_rate_d. (rad/s)) -> yaw_rate_d [-1,1]/1
  "Height controller "/1(Z_velocity_d (m/s)) -> Saturation2/1
  Saturation1/1 -> Demux/1
  Position controller/1(uxy) -> Saturation1/1
  Constant1/1 -> Z_velocity_d. [-1,1]/1
  Saturation2/1 -> Terminator/1

== system SIMULINK_U_a_C/control system_car1/Baseline Controller5 ==
  X_e : Inport
  Y_e : Inport  Port=2
  " Z_e " : Inport  Port=3
  Yaw_e : Inport  Port=4
  " V_x" : Inport  Port=5
  V_y : Inport  Port=6
  "V_z " : Inport  Port=7
  x_d : Inport  Port=8
  y_d : Inport  Port=9
  Z_d : Inport  Port=10
  Yaw_d : Inport  Port=11
  Constant : Constant  Commented=on  Value=omega*R*2
  Constant1 : Constant  Value=0
  Demux : Demux  Outputs=2
  Heading controller : Subsystem
  "Height controller " : Subsystem
  MATLAB Function : MATLAB Function  Commented=on  TreatAsAtomicUnit=on
  Position controller : Subsystem
  Saturation1 : Saturate  UpperLimit=lmt  LowerLimit=-lmt
  Saturation2 : Saturate  UpperLimit=lmt  LowerLimit=-lmt
  Terminator : Terminator
  ux : Outport  VectorParamsAs1DForOutWhenUnconnected=off
  uy : Outport  Port=2  VectorParamsAs1DForOutWhenUnconnected=off
  Z_velocity_d. [-1,1] : Outport  Port=3  VectorParamsAs1DForOutWhenUnconnected=off
  yaw_rate_d [-1,1] : Outport  Port=4  VectorParamsAs1DForOutWhenUnconnected=off
  wires:
  " Z_e "/1 -> "Height controller "/2(Z_e (m))
  X_e/1 -> Position controller/1(X_e (m))
  Y_e/1 -> Position controller/2(Y_e (m))
  Yaw_d/1 -> Heading controller/2(yaw_d. (rad))
  Demux/1 -> ux/1
  Demux/2 -> uy/1
  Constant/1 -> MATLAB Function/2(a)
  Z_d/1 -> "Height controller "/1(Z_d. (m))
  x_d/1 -> Position controller/3(X_d (m))
  y_d/1 -> Position controller/4(Y_d (m))
  Yaw_e/1 -> Heading controller/1(yaw_e (rad))  "yaw"
  "V_z "/1 -> "Height controller "/3(V_z)
  Heading controller/1(yaw_rate_d. (rad/s)) -> yaw_rate_d [-1,1]/1
  "Height controller "/1(Z_velocity_d (m/s)) -> Saturation2/1
  Saturation1/1 -> Demux/1
  Position controller/1(uxy) -> Saturation1/1
  Constant1/1 -> Z_velocity_d. [-1,1]/1
  Saturation2/1 -> Terminator/1

== system SIMULINK_U_a_C/control system_car1/Baseline Controller6 ==
  X_e : Inport
  Y_e : Inport  Port=2
  " Z_e " : Inport  Port=3
  Yaw_e : Inport  Port=4
  " V_x" : Inport  Port=5
  V_y : Inport  Port=6
  "V_z " : Inport  Port=7
  x_d : Inport  Port=8
  y_d : Inport  Port=9
  Z_d : Inport  Port=10
  Yaw_d : Inport  Port=11
  Constant : Constant  Commented=on  Value=omega*R*2
  Constant1 : Constant  Value=0
  Demux : Demux  Outputs=2
  Heading controller : Subsystem
  "Height controller " : Subsystem
  MATLAB Function : MATLAB Function  Commented=on  TreatAsAtomicUnit=on
  Position controller : Subsystem
  Saturation1 : Saturate  UpperLimit=lmt  LowerLimit=-lmt
  Saturation2 : Saturate  UpperLimit=lmt  LowerLimit=-lmt
  Terminator : Terminator
  ux : Outport  VectorParamsAs1DForOutWhenUnconnected=off
  uy : Outport  Port=2  VectorParamsAs1DForOutWhenUnconnected=off
  Z_velocity_d. [-1,1] : Outport  Port=3  VectorParamsAs1DForOutWhenUnconnected=off
  yaw_rate_d [-1,1] : Outport  Port=4  VectorParamsAs1DForOutWhenUnconnected=off
  wires:
  " Z_e "/1 -> "Height controller "/2(Z_e (m))
  X_e/1 -> Position controller/1(X_e (m))
  Y_e/1 -> Position controller/2(Y_e (m))
  Yaw_d/1 -> Heading controller/2(yaw_d. (rad))
  Demux/1 -> ux/1
  Demux/2 -> uy/1
  Constant/1 -> MATLAB Function/2(a)
  Z_d/1 -> "Height controller "/1(Z_d. (m))
  x_d/1 -> Position controller/3(X_d (m))
  y_d/1 -> Position controller/4(Y_d (m))
  Yaw_e/1 -> Heading controller/1(yaw_e (rad))  "yaw"
  "V_z "/1 -> "Height controller "/3(V_z)
  Heading controller/1(yaw_rate_d. (rad/s)) -> yaw_rate_d [-1,1]/1
  "Height controller "/1(Z_velocity_d (m/s)) -> Saturation2/1
  Saturation1/1 -> Demux/1
  Position controller/1(uxy) -> Saturation1/1
  Constant1/1 -> Z_velocity_d. [-1,1]/1
  Saturation2/1 -> Terminator/1

== system SIMULINK_U_a_C/control system_car1/Baseline Controller7 ==
  X_e : Inport
  Y_e : Inport  Port=2
  " Z_e " : Inport  Port=3
  Yaw_e : Inport  Port=4
  " V_x" : Inport  Port=5
  V_y : Inport  Port=6
  "V_z " : Inport  Port=7
  x_d : Inport  Port=8
  y_d : Inport  Port=9
  Z_d : Inport  Port=10
  Yaw_d : Inport  Port=11
  Constant : Constant  Commented=on  Value=omega*R*2
  Constant1 : Constant  Value=0
  Demux : Demux  Outputs=2
  Heading controller : Subsystem
  "Height controller " : Subsystem
  MATLAB Function : MATLAB Function  Commented=on  TreatAsAtomicUnit=on
  Position controller : Subsystem
  Saturation1 : Saturate  UpperLimit=lmt  LowerLimit=-lmt
  Saturation2 : Saturate  UpperLimit=lmt  LowerLimit=-lmt
  Terminator : Terminator
  ux : Outport  VectorParamsAs1DForOutWhenUnconnected=off
  uy : Outport  Port=2  VectorParamsAs1DForOutWhenUnconnected=off
  Z_velocity_d. [-1,1] : Outport  Port=3  VectorParamsAs1DForOutWhenUnconnected=off
  yaw_rate_d [-1,1] : Outport  Port=4  VectorParamsAs1DForOutWhenUnconnected=off
  wires:
  " Z_e "/1 -> "Height controller "/2(Z_e (m))
  X_e/1 -> Position controller/1(X_e (m))
  Y_e/1 -> Position controller/2(Y_e (m))
  Yaw_d/1 -> Heading controller/2(yaw_d. (rad))
  Demux/1 -> ux/1
  Demux/2 -> uy/1
  Constant/1 -> MATLAB Function/2(a)
  Z_d/1 -> "Height controller "/1(Z_d. (m))
  x_d/1 -> Position controller/3(X_d (m))
  y_d/1 -> Position controller/4(Y_d (m))
  Yaw_e/1 -> Heading controller/1(yaw_e (rad))  "yaw"
  "V_z "/1 -> "Height controller "/3(V_z)
  Heading controller/1(yaw_rate_d. (rad/s)) -> yaw_rate_d [-1,1]/1
  "Height controller "/1(Z_velocity_d (m/s)) -> Saturation2/1
  Saturation1/1 -> Demux/1
  Position controller/1(uxy) -> Saturation1/1
  Constant1/1 -> Z_velocity_d. [-1,1]/1
  Saturation2/1 -> Terminator/1

== system SIMULINK_U_a_C/control system_car1/Baseline Controller8 ==
  X_e : Inport
  Y_e : Inport  Port=2
  " Z_e " : Inport  Port=3
  Yaw_e : Inport  Port=4
  " V_x" : Inport  Port=5
  V_y : Inport  Port=6
  "V_z " : Inport  Port=7
  x_d : Inport  Port=8
  y_d : Inport  Port=9
  Z_d : Inport  Port=10
  Yaw_d : Inport  Port=11
  Constant : Constant  Commented=on  Value=omega*R*2
  Constant1 : Constant  Value=0
  Demux : Demux  Outputs=2
  Heading controller : Subsystem
  "Height controller " : Subsystem
  MATLAB Function : MATLAB Function  Commented=on  TreatAsAtomicUnit=on
  Position controller : Subsystem
  Saturation1 : Saturate  UpperLimit=lmt  LowerLimit=-lmt
  Saturation2 : Saturate  UpperLimit=lmt  LowerLimit=-lmt
  Terminator : Terminator
  ux : Outport  VectorParamsAs1DForOutWhenUnconnected=off
  uy : Outport  Port=2  VectorParamsAs1DForOutWhenUnconnected=off
  Z_velocity_d. [-1,1] : Outport  Port=3  VectorParamsAs1DForOutWhenUnconnected=off
  yaw_rate_d [-1,1] : Outport  Port=4  VectorParamsAs1DForOutWhenUnconnected=off
  wires:
  " Z_e "/1 -> "Height controller "/2(Z_e (m))
  X_e/1 -> Position controller/1(X_e (m))
  Y_e/1 -> Position controller/2(Y_e (m))
  Yaw_d/1 -> Heading controller/2(yaw_d. (rad))
  Demux/1 -> ux/1
  Demux/2 -> uy/1
  Constant/1 -> MATLAB Function/2(a)
  Z_d/1 -> "Height controller "/1(Z_d. (m))
  x_d/1 -> Position controller/3(X_d (m))
  y_d/1 -> Position controller/4(Y_d (m))
  Yaw_e/1 -> Heading controller/1(yaw_e (rad))  "yaw"
  "V_z "/1 -> "Height controller "/3(V_z)
  Heading controller/1(yaw_rate_d. (rad/s)) -> yaw_rate_d [-1,1]/1
  "Height controller "/1(Z_velocity_d (m/s)) -> Saturation2/1
  Saturation1/1 -> Demux/1
  Position controller/1(uxy) -> Saturation1/1
  Constant1/1 -> Z_velocity_d. [-1,1]/1
  Saturation2/1 -> Terminator/1

== system SIMULINK_U_a_C/control system_car1/Baseline Controller9 ==
  X_e : Inport
  Y_e : Inport  Port=2
  " Z_e " : Inport  Port=3
  Yaw_e : Inport  Port=4
  " V_x" : Inport  Port=5
  V_y : Inport  Port=6
  "V_z " : Inport  Port=7
  x_d : Inport  Port=8
  y_d : Inport  Port=9
  Z_d : Inport  Port=10
  Yaw_d : Inport  Port=11
  Constant : Constant  Commented=on  Value=omega*R*2
  Constant1 : Constant  Value=0
  Demux : Demux  Outputs=2
  Heading controller : Subsystem
  "Height controller " : Subsystem
  MATLAB Function : MATLAB Function  Commented=on  TreatAsAtomicUnit=on
  Position controller : Subsystem
  Saturation1 : Saturate  UpperLimit=lmt  LowerLimit=-lmt
  Saturation2 : Saturate  UpperLimit=lmt  LowerLimit=-lmt
  Terminator : Terminator
  ux : Outport  VectorParamsAs1DForOutWhenUnconnected=off
  uy : Outport  Port=2  VectorParamsAs1DForOutWhenUnconnected=off
  Z_velocity_d. [-1,1] : Outport  Port=3  VectorParamsAs1DForOutWhenUnconnected=off
  yaw_rate_d [-1,1] : Outport  Port=4  VectorParamsAs1DForOutWhenUnconnected=off
  wires:
  " Z_e "/1 -> "Height controller "/2(Z_e (m))
  X_e/1 -> Position controller/1(X_e (m))
  Y_e/1 -> Position controller/2(Y_e (m))
  Yaw_d/1 -> Heading controller/2(yaw_d. (rad))
  Demux/1 -> ux/1
  Demux/2 -> uy/1
  Constant/1 -> MATLAB Function/2(a)
  Z_d/1 -> "Height controller "/1(Z_d. (m))
  x_d/1 -> Position controller/3(X_d (m))
  y_d/1 -> Position controller/4(Y_d (m))
  Yaw_e/1 -> Heading controller/1(yaw_e (rad))  "yaw"
  "V_z "/1 -> "Height controller "/3(V_z)
  Heading controller/1(yaw_rate_d. (rad/s)) -> yaw_rate_d [-1,1]/1
  "Height controller "/1(Z_velocity_d (m/s)) -> Saturation2/1
  Saturation1/1 -> Demux/1
  Position controller/1(uxy) -> Saturation1/1
  Constant1/1 -> Z_velocity_d. [-1,1]/1
  Saturation2/1 -> Terminator/1

== system SIMULINK_U_a_C/plot/Subsystem ==
  Constant : Constant  Value=fixed_step_size
  Constant1 : Constant  Value=XMIN
  Constant10 : Constant  Value=b
  Constant11 : Constant  Value=k
  Constant12 : Constant  Value=bb
  Constant13 : Constant  Value=w1
  Constant14 : Constant  Value=w2
  Constant2 : Constant  Value=XMAX
  Constant3 : Constant  Value=YMIN
  Constant4 : Constant  Value=YMAX
  Constant5 : Constant  Value=ZMIN
  Constant6 : Constant  Value=ZMAX
  Constant7 : Constant  Value=draw_gif
  Constant8 : Constant  Value=act_end
  Constant9 : Constant  Value=a
  step_time : Outport  VectorParamsAs1DForOutWhenUnconnected=off
  act_end : Outport  Port=2  VectorParamsAs1DForOutWhenUnconnected=off
  x_min : Outport  Port=3  VectorParamsAs1DForOutWhenUnconnected=off
  x_max : Outport  Port=4  VectorParamsAs1DForOutWhenUnconnected=off
  y_min : Outport  Port=5  VectorParamsAs1DForOutWhenUnconnected=off
  y_max : Outport  Port=6  VectorParamsAs1DForOutWhenUnconnected=off
  z_min : Outport  Port=7  VectorParamsAs1DForOutWhenUnconnected=off
  z_max : Outport  Port=8  VectorParamsAs1DForOutWhenUnconnected=off
  a : Outport  Port=9  VectorParamsAs1DForOutWhenUnconnected=off
  b : Outport  Port=10  VectorParamsAs1DForOutWhenUnconnected=off
  k : Outport  Port=11  VectorParamsAs1DForOutWhenUnconnected=off
  bb : Outport  Port=12  VectorParamsAs1DForOutWhenUnconnected=off
  w1 : Outport  Port=13  VectorParamsAs1DForOutWhenUnconnected=off
  w2 : Outport  Port=14  VectorParamsAs1DForOutWhenUnconnected=off
  draw_gif : Outport  Port=15  VectorParamsAs1DForOutWhenUnconnected=off
  wires:
  Constant/1 -> step_time/1
  Constant1/1 -> x_min/1
  Constant2/1 -> x_max/1
  Constant3/1 -> y_min/1
  Constant4/1 -> y_max/1
  Constant7/1 -> draw_gif/1
  Constant6/1 -> z_max/1
  Constant5/1 -> z_min/1
  Constant13/1 -> w1/1
  Constant10/1 -> b/1
  Constant9/1 -> a/1
  Constant14/1 -> w2/1
  Constant11/1 -> k/1
  Constant8/1 -> act_end/1
  Constant12/1 -> bb/1

== system SIMULINK_U_a_C/send_ctrl_signal_UAV/Send Command 1 ==
  pos : Inport
  u : Inport  Port=2
  Bus Selector : BusSelector  OutputSignals=droneyeeUAV1_states.x,droneyeeUAV1_states.y  OutputAsBus=on
  Bus Selector1 : BusSelector  OutputSignals=uav1.u_vx,uav1.u_vy,uav1.u_vz,uav1.u_rate_roll,uav1.u_rate_pitch,uav1.u_rate_yaw
  Clock : Clock
  Compare To Constant : simulink/Logic and Bit Operations/Compare To Constant  relop=>=  const=0.1  OutDataTypeStr=boolean
  Constant : Constant  Value=sim_end_time
  Constant1 : Constant  Value=0
  Constant2 : Constant  Value=uav1num
  Constant3 : Constant  Value=Vel_Switch_1
  Constant4 : Constant  Value=0
  Constant5 : Constant  Value=0
  K : Gain
  K1 : Gain
  K2 : Gain
  Logical Operator : Logic  Inputs=3  AllPortsSameDT=off  OutDataTypeStr=boolean
  Mux : Mux  Inputs=8
  Mux1 : Mux  Inputs=5
  Subsystem : Subsystem
  Sum : Sum  Inputs=|-+
  Switch{1..3,6,12} (5 alike) : Switch  Criteria=u2 > Threshold  Threshold=0.001  SaturateOnIntegerOverflow=off  InputSameDT=off
  Switch4 : Switch  Criteria=u2 > Threshold  SaturateOnIntegerOverflow=off  InputSameDT=off
  Switch5 : Switch  Criteria=u2 > Threshold  SaturateOnIntegerOverflow=off  InputSameDT=off
  uav1 : Constant  Value=0
  tag scope: copterSend1=global, mode1=global, sim_CopterSend1=global
  wires:
  Constant1/1 -> Switch3/3, Switch2/3, Switch1/3, Switch12/3
  K1/1 -> Mux1/5, Mux/7
  Switch1/1 -> K/1
  Bus Selector1/2 -> Switch1/1  "<u_vy>"
  Switch2/1 -> K2/1
  Bus Selector1/3 -> Switch2/1  "<u_vz>"
  Switch3/1 -> K1/1
  Logical Operator/1 -> Switch1/2, Switch12/2, Switch2/2, Switch3/2
  K2/1 -> Mux1/4, Mux/4
  Clock/1 -> Sum/1
  Constant/1 -> Sum/2
  Sum/1 -> Compare To Constant/1
  Compare To Constant/1 -> Logical Operator/2
  pos/1 -> Bus Selector/1
  Bus Selector/1 -> Subsystem/1(In1)
  u/1 -> Bus Selector1/1
  Bus Selector1/1 -> Switch12/1  "<u_vx>"
  Bus Selector1/6 -> Switch3/1  "<u_rate_yaw>"
  Bus Selector1/4 -> Mux/5  "<u_rate_roll>"
  Bus Selector1/5 -> Mux/6  "<u_rate_pitch>"
  Constant2/1 -> Mux/1
  Constant3/1 -> Logical Operator/3
  Switch12/1 -> Mux1/2, Mux/2
  K/1 -> Mux1/3, Mux/3
  Switch6/1 -> Mux/8
  Subsystem/1(Out1) -> Logical Operator/1
  Constant4/1 -> Mux1/1
  Switch4/1 -> [sim_CopterSend1]
  Mux1/1 -> Switch4/3
  Mux/1 -> Switch5/1
  Switch5/1 -> [copterSend1]
  [sim_flag] -> Switch5/2, Switch4/2
  Constant5/1 -> [mode1]
  uav1/1 -> Switch6/3
  [mode1] -> Switch6/2, Switch6/1

== system SIMULINK_U_a_C/send_ctrl_signal_UAV/Send Command 10 ==
  pos : Inport
  u : Inport  Port=2
  Bus Selector : BusSelector  OutputSignals=x,y  OutputAsBus=on
  Bus Selector1 : BusSelector  OutputSignals=u_vx,u_vy,u_vz,u_rate_roll,u_rate_pitch,u_rate_yaw
  Clock : Clock
  Compare To Constant : simulink/Logic and Bit Operations/Compare To Constant  relop=>=  const=0.1  OutDataTypeStr=boolean
  Constant : Constant  Value=sim_end_time
  Constant1 : Constant  Value=0
  Constant2 : Constant  Value=uav10num
  Constant3 : Constant  Value=Vel_Switch_10
  Constant4 : Constant  Value=0
  K : Gain
  K1 : Gain
  K2 : Gain
  Logical Operator : Logic  Inputs=3  AllPortsSameDT=off  OutDataTypeStr=boolean
  Mux : Mux  Inputs=8
  Mux1 : Mux  Inputs=5
  Subsystem : Subsystem
  Sum : Sum  Inputs=|-+
  Switch{1..3,6,12} (5 alike) : Switch  Criteria=u2 > Threshold  Threshold=0.001  SaturateOnIntegerOverflow=off  InputSameDT=off
  Switch4 : Switch  Criteria=u2 > Threshold  SaturateOnIntegerOverflow=off  InputSameDT=off
  Switch5 : Switch  Criteria=u2 > Threshold  SaturateOnIntegerOverflow=off  InputSameDT=off
  uav10 : Constant
  tag scope: copterSend10=global, sim_CopterSend10=global
  wires:
  Constant1/1 -> Switch3/3, Switch2/3, Switch1/3, Switch12/3
  K1/1 -> Mux1/5, Mux/7
  Switch1/1 -> K/1
  Bus Selector1/2 -> Switch1/1  "<u_vy>"
  Switch2/1 -> K2/1
  Bus Selector1/3 -> Switch2/1  "<u_vz>"
  Switch3/1 -> K1/1
  Logical Operator/1 -> Switch1/2, Switch12/2, Switch2/2, Switch3/2
  K2/1 -> Mux1/4, Mux/4
  Clock/1 -> Sum/1
  Constant/1 -> Sum/2
  Sum/1 -> Compare To Constant/1
  Compare To Constant/1 -> Logical Operator/2
  pos/1 -> Bus Selector/1
  Bus Selector/1 -> Subsystem/1(In1)
  u/1 -> Bus Selector1/1
  Bus Selector1/1 -> Switch12/1  "<u_vx>"
  Bus Selector1/6 -> Switch3/1  "<u_rate_yaw>"
  Bus Selector1/4 -> Mux/5  "<u_rate_roll>"
  Bus Selector1/5 -> Mux/6  "<u_rate_pitch>"
  Constant2/1 -> Mux/1
  Constant3/1 -> Logical Operator/3
  Switch12/1 -> Mux1/2, Mux/2
  K/1 -> Mux1/3, Mux/3
  Switch6/1 -> Mux/8
  Subsystem/1(Out1) -> Logical Operator/1
  Constant4/1 -> Mux1/1
  Switch4/1 -> [sim_CopterSend10]
  Mux1/1 -> Switch4/3
  Mux/1 -> Switch5/1
  Switch5/1 -> [copterSend10]
  [sim_flag] -> Switch5/2, Switch4/2
  uav10/1 -> Switch6/3
  [mode1] -> Switch6/2, Switch6/1
